simulink model "AME552_HW2_P4_SimulinkModel"  (R2024b)
settings: Solver=VariableStepAuto  StartTime=0.0  StopTime=5  RelTol=1e-3
values from neighbouring files (symbols this model uses):
  A = 1    [AME552_HW2_P4.m]    (also in AME552_HW2_P4_Simulink.m)
  B = 1    [AME552_HW2_P4.m]    (also in AME552_HW2_P4_Simulink.m)
  de0 = de0_space(j)    [AME552_HW2_P4_Simulink.m]
  J = 1    [AME552_HW2_P4.m]    (also in AME552_HW2_P4_Simulink.m)
  kb = 1    [AME552_HW2_P4.m]    (also in AME552_HW2_P4_Simulink.m)
  ki = 2    [AME552_HW2_P4.m]    (also in AME552_HW2_P4_Simulink.m)
  kp = 1    [AME552_HW2_P4.m]    (also in AME552_HW2_P4_Simulink.m)
  wc = 0.5    [AME552_HW2_P4.m]    (also in AME552_HW2_P4_Simulink.m = 0.1)
libraries: simulink x1
settings Model: Creator=lewis  LastModifiedBy=lewis

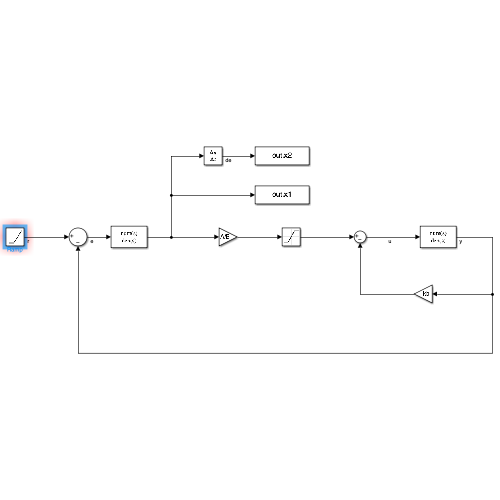
[thumbnail: Simulink's stored preview of the top-level diagram]
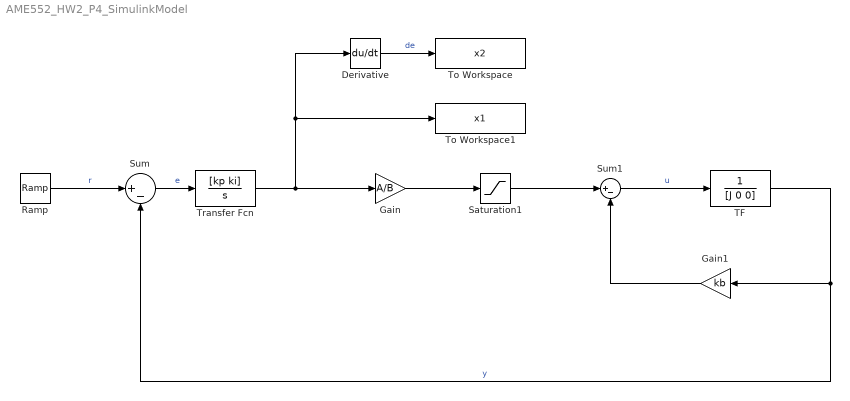
== system AME552_HW2_P4_SimulinkModel ==
  Derivative : Derivative
  Gain : Gain  Gain=A/B
  Gain1 : Gain  Gain=kb
  Ramp : simulink/Sources/Ramp  slope=de0  start=0  InitialOutput=e0+wc
  Saturation1 : Saturate  UpperLimit=A  LowerLimit=-A
  Sum : Sum  Inputs=|+-
  Sum1 : Sum  Inputs=|+-
  TF : TransferFcn  Denominator=[J 0 0]
  To Workspace : ToWorkspace  VariableName=x2  SaveFormat=Timeseries  SampleTime=-1
  To Workspace1 : ToWorkspace  VariableName=x1  SaveFormat=Timeseries  SampleTime=-1
  Transfer Fcn : TransferFcn  Numerator=[kp ki]  Denominator=[1 0]
  wires:
  Sum/1 -> Transfer Fcn/1  "e"
  TF/1 -> Gain1/1, Sum/2  "y"
  Derivative/1 -> To Workspace/1  "de"
  Sum1/1 -> TF/1  "u"
  Gain1/1 -> Sum1/2
  Ramp/1 -> Sum/1  "r"
  Transfer Fcn/1 -> Gain/1, To Workspace1/1, Derivative/1
  Gain/1 -> Saturation1/1
  Saturation1/1 -> Sum1/1
